simulink model "suspmodel"  (Simulink 2.00)
settings: Solver=ode45  StartTime=0.0  StopTime=50  RelTol=1e-3  AbsTol=1e-6
values from neighbouring files (symbols this model uses):
  b1 = 350    [setup_suspension.m]
  b2 = 15020    [setup_suspension.m]
undefined symbols (not defined in the file or in its folder): k1, k2, m1, m2
settings Model: ConsistencyChecking=off

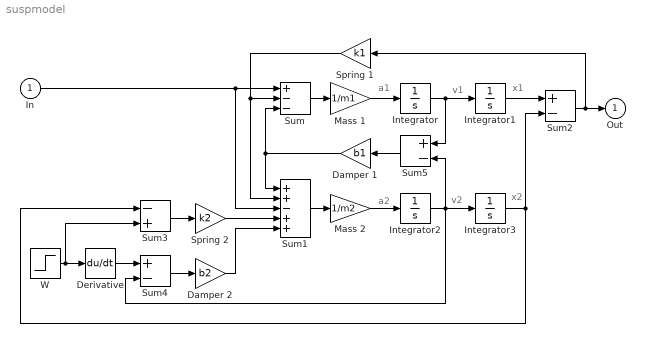
== system suspmodel ==
  note: a1
  note: v1
  note: x1
  note: a2
  note: v2
  note: x2
  In : Inport  Port=1  PortWidth=-1  SampleTime=-1
  Damper 1 : Gain  Orientation=left  Gain=b1
  Damper 2 : Gain  Gain=b2
  Derivative : Derivative
  Integrator{,1..3} (4 alike) : Integrator  ExternalReset=none  InitialConditionSource=internal  InitialCondition=0  LimitOutput=off  UpperSaturationLimit=inf  LowerSaturationLimit=-inf  ShowSaturationPort=off  ShowStatePort=off  AbsoluteTolerance=auto
  Mass 1 : Gain  Gain=1/m1
  Mass 2 : Gain  Gain=1/m2
  Spring 1 : Gain  Orientation=left  Gain=k1
  Spring 2 : Gain  Gain=k2
  Sum : Sum  Inputs=+--
  Sum1 : Sum  Inputs=++-++
  Sum2 : Sum  Inputs=+-
  Sum3 : Sum  Inputs=-+
  Sum4 : Sum  Inputs=+-
  Sum5 : Sum  Orientation=left  Inputs=+-
  W : Step  Time=0  Before=0  After=0
  Out : Outport  Port=1  InitialOutput=0
  wires:
  Mass 2/1 -> Integrator2/1
  Sum1/1 -> Mass 2/1
  Integrator2/1 -> Integrator3/1, Sum4/2, Sum5/2
  Sum5/1 -> Damper 1/1
  Damper 1/1 -> Sum1/1, Sum/3
  Mass 1/1 -> Integrator/1
  Sum/1 -> Mass 1/1
  Integrator1/1 -> Sum2/1
  Integrator/1 -> Integrator1/1, Sum5/1
  Integrator3/1 -> Sum2/2, Sum3/1
  Sum2/1 -> Spring 1/1, Out/1
  Spring 1/1 -> Sum/2, Sum1/2
  Damper 2/1 -> Sum1/5
  Spring 2/1 -> Sum1/4
  Sum3/1 -> Spring 2/1
  Sum4/1 -> Damper 2/1
  In/1 -> Sum/1, Sum1/3
  Derivative/1 -> Sum4/1
  W/1 -> Sum3/2, Derivative/1
